simulink model "project1_week2"  (R2021a)
settings: Solver=VariableStepAuto  StartTime=0.0  StopTime=inf  RelTol=1e-3
settings Model: EnablePacing=on  PacingRate=0.320000  Creator=RASIKA MALGI  LastModifiedBy=RASIKA MALGI
settings SolverCC: AlgebraicLoopSolver=TrustRegion
settings DebuggingCC: SFMachineParentedDataDiag=warning

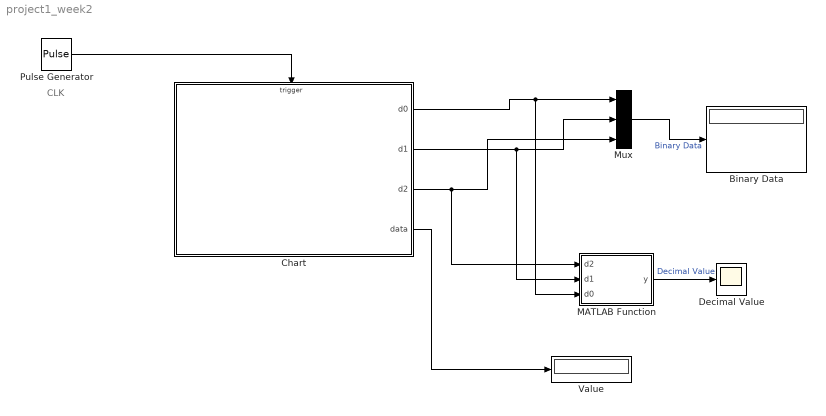
== system project1_week2 ==
  note: CLK
  Binary Data : Display
  Chart : Stateflow chart  TreatAsAtomicUnit=on
  Decimal Value : Scope
  MATLAB Function : MATLAB Function  TreatAsAtomicUnit=on
  Mux : Mux  Inputs=3
  Pulse Generator : DiscretePulseGenerator  PulseType=Time based  Period=0.5  PulseWidth=5
  Value : Display
  wires:
  Chart/1(d0) -> MATLAB Function/3(d0), Mux/1
  Chart/2(d1) -> MATLAB Function/2(d1), Mux/2
  Chart/3(d2) -> MATLAB Function/1(d2), Mux/3
  Chart/4(data) -> Value/1
  Pulse Generator/1 -> Chart/Trigger
  Mux/1 -> Binary Data/1  "Binary Data"
  MATLAB Function/1(y) -> Decimal Value/1  "Decimal Value"

== matlab function project1_week2/MATLAB Function ==
  data: d2 input; y output; d1 input; d0 input
function y= fcn(d2,d1,d0)
if(d2==0 && d1==0 && d0==0)
    y=0;
elseif(d2==0 && d1==0 && d0==1)
    y=1;
elseif(d2==0 && d1==1 && d0==0)
    y=2;
elseif(d2==0 && d1==1 && d0==1)
    y=3;
elseif(d2==1 && d1==0 && d0==0)
    y=4;
else
    y=0;
    
end

== stateflow chart project1_week2/Chart ==
  settings: executeAtInitialization=1
  state ConversionState [parallel]
    during:
    data2=d2;
    data1=d1;
    data0=d0;
    r=0;
    check(data2,data1,data0);
    settings: executionOrder=1
  state digit0 [parallel]
    settings: executionOrder=2
    state digit_zero
      entry:
      d0=0;
    state digit_one
      entry:
      d0=1;
    digit0.digit_one -> digit0.digit_zero [order 2] : [r==1]
    (default) -> digit0.digit_zero
    digit0.digit_one -> digit0.digit_zero [order 1] : pulse{send(inc1);}
    digit0.digit_zero -> digit0.digit_one : pulse
  note: 000-0
      | 001-1
      | 010-2
      | 011-3
      | 100-4
      | 101-5
      | 110-6
      | 111-7
  state check(d02,d01,d00) [function]
    (default) -> (junction 22) : % Conversion to Decimal
    (junction 22) -> (junction 69) [order 1] : [d02==0 && d01==0 && d00==0]
    (junction 22) -> (junction 54) [order 2]
    (junction 69) -> (junction 46) : {data=0;
        | r=0;}
    (junction 54) -> (junction 31) [order 1] : [d02==0 && d01==0 && d00==1]
    (junction 54) -> (junction 29) [order 2]
    (junction 31) -> (junction 27) : {data=1;
        | r=0;}
    (junction 29) -> (junction 59) [order 1] : [d02==0 && d01==1 && d00==0]
    (junction 29) -> (junction 42) [order 2]
    (junction 59) -> (junction 61) : {data=2;
        | r=0;}
    (junction 42) -> (junction 26) [order 1] : [d02==0 && d01==1 && d00==1]
    (junction 42) -> (junction 43) [order 2]
    (junction 26) -> (junction 41) : {data=3;
        | r=0;}
    (junction 43) -> (junction 68) [order 1] : [d02==1 && d01==0 && d00==0]
    (junction 43) -> (junction 60) [order 2]
    (junction 68) -> (junction 44) : {data=4;
        | r=0;}
    (junction 44) -> (junction 60)
    (junction 41) -> (junction 44)
    (junction 61) -> (junction 41)
    (junction 27) -> (junction 61)
    (junction 46) -> (junction 27)
    (junction 60) -> (junction 64)
  state digit1 [parallel]
    settings: executionOrder=3
    state digit_zero
      entry:
      d1=0;
    state digit_one
      entry:
      d1=1;
    (default) -> digit1.digit_zero
    digit1.digit_one -> digit1.digit_zero : inc1{send(inc2);}
    digit1.digit_zero -> digit1.digit_one : inc1
  state digit2 [parallel]
    settings: executionOrder=4
    state digit_zero
      entry:
      d2=0;
    state digit_one
      entry:
      d2=1;
    (default) -> digit2.digit_zero
    digit2.digit_one -> digit2.digit_zero : inc2
    digit2.digit_zero -> digit2.digit_one : inc2
  (default) -> digit0
  data: d02 function_input; d01 function_input; d00 function_input; d0 output =1; d1 output =1; d2 output =1; data0 local =1; data1 local =1; data2 local; r local =0; data output =4
  events: pulse input RISING_EDGE_EVENT; inc1 local FUNCTION_CALL_EVENT; inc2 local FUNCTION_CALL_EVENT
